simulink model "Moteur1_v2"  (R2021a)
settings: Solver=VariableStepAuto  StartTime=0.0  StopTime=100  RelTol=1e-3
model workspace (MAT data in the model file):
  Kfcem = 0.00109
  L = 1e-06
  R = 3.18
  VPwm = 12
  wm = 1000
settings Model: Creator=Jetr1804  LastModifiedBy=Jetr1804

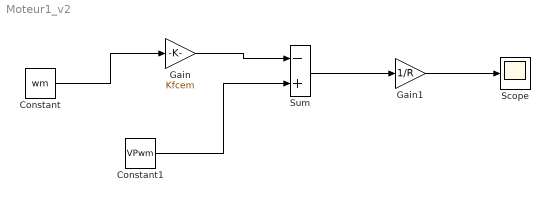
== system Moteur1_v2 ==
  Constant : Constant  Value=wm
  Constant1 : Constant  Value=VPwm
  Gain : Gain  Gain=Kfcem
  Gain1 : Gain  Gain=1/R
  Scope : Scope
  Sum : Sum  Inputs=-+
  wires:
  Constant/1 -> Gain/1
  Gain/1 -> Sum/1
  Constant1/1 -> Sum/2
  Sum/1 -> Gain1/1
  Gain1/1 -> Scope/1
